simulink model "FOC"  (R2026a)
settings: Solver=FixedStepDiscrete  StopTime=inf  FixedStep=Ts  EnableMultiTasking=on
InitFcn:
  | ParameterInit
undefined symbols (not defined in the file): drive, FAKF, motor, Ts
libraries: mcbhdlcontrolslib x9, matrix_library x8, simulink x7, mcbcontrolslib x5, mcbsensorlessestimatorlib x2, mcbeeMathTransformLib x2, slpidlib x2, mcbpositiondecoderlib x1, sl_discontinuities x1
(part 1 of 2)
settings Model: Creator=xueji  LastModifiedBy=xuejf
settings DataIOCC: SaveFormat=StructureWithTime
settings OptimizationCC: ConditionallyExecuteInputs=off  UseDivisionForNetSlopeComputation=on  GainParamInheritBuiltInType=on  UseFloatMulNetSlope=on  StrengthReduction=on  NoFixptDivByZeroProtection=on  EfficientFloat2IntCast=on  OptimizationPriority=Speed  MultiThreadedLoops=on  AutoScheduleForLoops=on  UseRestrictQualifier=on
settings DebuggingCC: ParameterOverflowMsg=none  ParameterUnderflowMsg=error  ParameterPrecisionLossMsg=none
settings HardwareCC: ProdLargestAtomicInteger=Long  ProdLargestAtomicFloat=Double  ProdHWDeviceType=ARM Compatible->ARM Cortex  TargetBitPerPointer=64.0  TargetBitPerSizeT=64.0  TargetBitPerPtrDiffT=64.0  TargetLongLongMode=on  TargetIntDivRoundTo=Zero  TargetEndianess=LittleEndian  TargetWordSize=64.0  TargetHWDeviceType=MATLAB Host  ProdEqTarget=off
settings SFSimCC: SimTargetLang=C++
settings RTWCC: SystemTargetFile=ert.tlc  GenCodeOnly=on  Toolchain=GNU Tools for ARM Embedded Processors  BuildConfiguration=Faster Runs  DataTypeReplacement=CDataTypesFixedWidth  Description=Embedded Coder
settings CodeAppCC: CustomSymbolStrGlobalVar=rt$N$M  CustomSymbolStrType=$N$M  CustomSymbolStrFcn=$N$M$F  CustomSymbolStrMacro=$N$M  MATLABSourceComments=on  UseSimReservedNames=on
settings ERTTargetCC: ExtModeTransport=1.0  ExtModeMexFile=ext_serial_win32_comm  RootIOFormat=Structure reference  ERTFilePackagingFormat=Compact  MaxIdInt64=INT64_MAX  MinIdInt64=INT64_MIN  MaxIdUint64=UINT64_MAX  MaxIdInt32=INT32_MAX  MinIdInt32=INT32_MIN  MaxIdUint32=UINT32_MAX  MaxIdInt16=INT16_MAX  MinIdInt16=INT16_MIN  MaxIdUint16=UINT16_MAX  MaxIdInt8=INT8_MAX  MinIdInt8=INT8_MIN  MaxIdUint8=UINT8_MAX  GenerateSampleERTMain=on  CombineOutputUpdateFcns=off  SupportAbsoluteTime=off  PreserveMATLABNamespacesInGeneratedCode=off  CodeInterfacePackaging=Reusable function  SupportComplex=off
settings SimscapeCC: SimscapeNominalValues="[{\"value\":\"1\",\"unit\":\"A\"},{\"value\":\"1\",\"unit\":\"bar\"},{\"value\":\"1\",\"unit\":\"cm^2\"},{\"value\":\"1\",\"unit\":\"cm^3/s\"},{\"value\":\"1\",\"unit\":\"kJ/kg\"},{\"value\":\"1\",\"unit\":\"kW\"},{\"value\":\"1\",\"unit\":\"l\"},{\"value\":\"1\",\"unit\":\"N\"},{\"value\":\"1\",\"unit\":\"N*m\"},{\"value\":\"1\",\"unit\":\"V\"}]"  SimscapeLogType=none  SimscapeLogDataHistory=5000.0

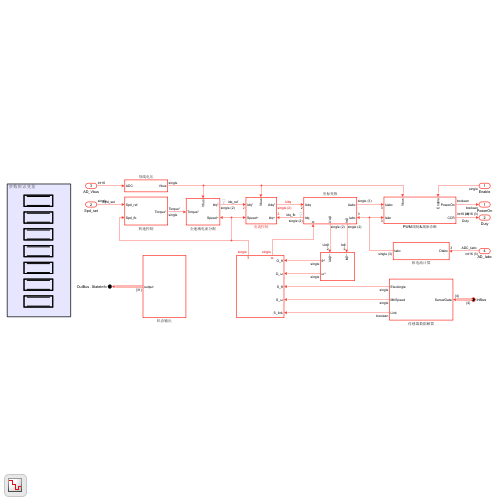
[thumbnail: Simulink's stored preview of the top-level diagram]
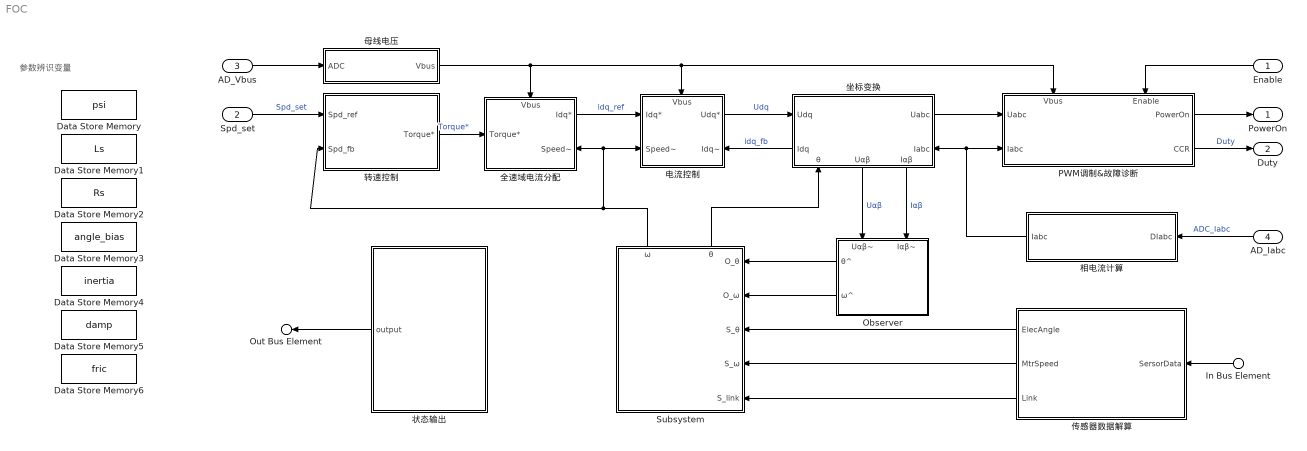
== system FOC ==
  note: 参数辨识变量
  Enable : Inport  OutDataTypeStr=single  PortDimensions=1  SampleTime=[5.0000000000000002e-05,0]
  Spd_set : Inport  Port=2  OutDataTypeStr=single  PortDimensions=1  SampleTime=[5.0000000000000002e-05,0]
  AD_Vbus : Inport  Port=3  OutDataTypeStr=int16  PortDimensions=1  SampleTime=[5.0000000000000002e-05,0]
  AD_Iabc : Inport  Port=4  OutDataTypeStr=int16  PortDimensions=3  SampleTime=[5.0000000000000002e-05,0]
  In Bus Element : Inport  Port=5  PortName=InBus
  Data Store Memory : DataStoreMemory  DataStoreName=psi  WriteAfterWriteMsg=warning  ShowAdditionalParam=off
  Data Store Memory1 : DataStoreMemory  DataStoreName=Ls  WriteAfterWriteMsg=warning  ShowAdditionalParam=off
  Data Store Memory2 : DataStoreMemory  DataStoreName=Rs  WriteAfterWriteMsg=warning  ShowAdditionalParam=off
  Data Store Memory3 : DataStoreMemory  DataStoreName=angle_bias  WriteAfterWriteMsg=warning  ShowAdditionalParam=off  OutDataTypeStr=single
  Data Store Memory4 : DataStoreMemory  DataStoreName=inertia  WriteAfterWriteMsg=warning  ShowAdditionalParam=off  OutDataTypeStr=single
  Data Store Memory5 : DataStoreMemory  DataStoreName=damp  WriteAfterWriteMsg=warning  ShowAdditionalParam=off  OutDataTypeStr=single
  Data Store Memory6 : DataStoreMemory  DataStoreName=fric  WriteAfterWriteMsg=warning  ShowAdditionalParam=off  OutDataTypeStr=single
  Observer : Subsystem
      settings: MinAlgLoopOccurrences=on  PortSchema="{\"entries\":[{\"content\":{\"sides\":[{\"content\":{\"connectorIds\":[\"Out1\",\"Out2\"]},\"type\":\"ConnectorPlacement.EquallySpacedRectSide\",\"uuid\":\"e0bc5786-ce1d-4855-a3b5-736cd4452aa5\"},{\"content\":{\"side\":\"RIGHT\"},\"type\":\"ConnectorPlacement.EquallySpacedRectSide\",\"uuid\":\"2fd42ec2-cdfa-4ba6-bbae-150322a5d493\"},{\"content\":{\"connectorIds\":[\"In1\",\"In2\"],\"side\":\"TOP\"},\"type\":\"ConnectorPlacement.EquallySpacedRectSide\",\"uuid\":\"b90c8681-3a82-4d31-b956-3e10c61bd992\"}]},\"type\":\"ConnectorPlacement.EquallySpacedConnector\",\"uuid\":\"5605c3b5-9268-4421-a61a-19e31e78b2b2\"}],\"packageUris\":[\"http://schema.mathworks.com/mf0/Connector/R2020b\"],\"version\":\"1.0\"}"
  PWM调制&故障诊断 : Subsystem
      settings: PortSchema="{\"entries\":[{\"content\":{\"sides\":[{\"content\":{\"connectorIds\":[\"In1\",\"In2\"]},\"type\":\"ConnectorPlacement.EquallySpacedRectSide\",\"uuid\":\"492d6452-e717-42c4-995f-3faa38429cae\"},{\"content\":{\"connectorIds\":[\"Out1\",\"Out2\"],\"side\":\"RIGHT\"},\"type\":\"ConnectorPlacement.EquallySpacedRectSide\",\"uuid\":\"a45b9f70-76fb-43db-a233-80127821733d\"},{\"content\":{\"connectorIds\":[\"In3\",\"In4\"],\"side\":\"TOP\"},\"type\":\"ConnectorPlacement.EquallySpacedRectSide\",\"uuid\":\"87480e42-0fd9-4078-9596-9cf4a8d8a61b\"},{\"content\":{\"side\":\"BOTTOM\"},\"type\":\"ConnectorPlacement.EquallySpacedRectSide\",\"uuid\":\"e85548a5-948a-4384-9ce6-748091ec18d7\"}]},\"type\":\"ConnectorPlacement.EquallySpacedConnector\",\"uuid\":\"18d7a9be-c392-4737-8548-f782ad0f8f26\"}],\"packageUris\":[\"http://schema.mathworks.com/mf0/Connector/R2020b\"],\"version\":\"1.0\"}"
  Subsystem : Subsystem
      settings: PortSchema="{\"entries\":[{\"content\":{\"sides\":[{\"content\":{},\"type\":\"ConnectorPlacement.EquallySpacedRectSide\",\"uuid\":\"d4a4fcc6-9eab-45aa-b231-b7af833cd8c6\"},{\"content\":{\"connectorIds\":[\"In1\",\"In2\",\"In3\",\"In4\",\"In5\"],\"side\":\"RIGHT\"},\"type\":\"ConnectorPlacement.EquallySpacedRectSide\",\"uuid\":\"bf374db6-391b-4179-b18d-5bc8f845fc33\"},{\"content\":{\"connectorIds\":[\"Out1\",\"Out2\"],\"side\":\"TOP\"},\"type\":\"ConnectorPlacement.EquallySpacedRectSide\",\"uuid\":\"b7b6826e-7c33-41ba-b3c7-d16a7d7beb3a\"}]},\"type\":\"ConnectorPlacement.EquallySpacedConnector\",\"uuid\":\"61c6cbd8-a55e-4c51-8b84-52df934ee1be\"}],\"packageUris\":[\"http://schema.mathworks.com/mf0/Connector/R2020b\"],\"version\":\"1.0\"}"
  传感器数据解算 : Subsystem
  全速域电流分配 : Subsystem
      settings: PortSchema="{\"entries\":[{\"content\":{\"sides\":[{\"content\":{\"connectorIds\":[\"In1\"]},\"type\":\"ConnectorPlacement.EquallySpacedRectSide\",\"uuid\":\"55c1d0af-1e12-4135-aa70-ca0befd6bb29\"},{\"content\":{\"connectorIds\":[\"Out1\",\"In3\"],\"side\":\"RIGHT\"},\"type\":\"ConnectorPlacement.EquallySpacedRectSide\",\"uuid\":\"d5856c39-d2d9-42bf-88a6-12c62f6eb837\"},{\"content\":{\"connectorIds\":[\"In2\"],\"side\":\"TOP\"},\"type\":\"ConnectorPlacement.EquallySpacedRectSide\",\"uuid\":\"f04465a3-695d-494e-bf21-7b8ba0e1a298\"}]},\"type\":\"ConnectorPlacement.EquallySpacedConnector\",\"uuid\":\"e6412d78-9d8b-45ef-81b3-23a4fb87ae10\"}],\"packageUris\":[\"http://schema.mathworks.com/mf0/Connector/R2020b\"],\"version\":\"1.0\"}"
  坐标变换 : Subsystem
      settings: PortSchema="{\"entries\":[{\"content\":{\"sides\":[{\"content\":{\"connectorIds\":[\"In1\",\"Out4\"]},\"type\":\"ConnectorPlacement.EquallySpacedRectSide\",\"uuid\":\"19423b74-9855-4da1-a32f-fc09d117de38\"},{\"content\":{\"connectorIds\":[\"Out1\",\"In3\"],\"side\":\"RIGHT\"},\"type\":\"ConnectorPlacement.EquallySpacedRectSide\",\"uuid\":\"45d897d7-b2dc-4681-bc4b-90a4bd929118\"},{\"content\":{\"connectorIds\":[],\"side\":\"TOP\"},\"type\":\"ConnectorPlacement.EquallySpacedRectSide\",\"uuid\":\"59354a96-0169-49af-a302-86e785c620a3\"},{\"content\":{\"connectorIds\":[\"In2\",\"Out2\",\"Out3\"],\"side\":\"BOTTOM\"},\"type\":\"ConnectorPlacement.EquallySpacedRectSide\",\"uuid\":\"fb332ee8-d153-4216-8303-19cfa3862110\"}]},\"type\":\"ConnectorPlacement.EquallySpacedConnector\",\"uuid\":\"5f6d72a6-e6b8-48f2-bb88-1ad3720f15b2\"}],\"packageUris\":[\"http://schema.mathworks.com/mf0/Connector/R2020b\"],\"version\":\"1.0\"}"
  母线电压 : Subsystem
  状态输出 : Subsystem
      settings: PortSchema="{\"entries\":[{\"content\":{\"sides\":[{\"content\":{\"connectorIds\":[\"Out1\"]},\"type\":\"ConnectorPlacement.EquallySpacedRectSide\",\"uuid\":\"5ecb5947-9baa-4bfe-8641-96ff20667d62\"},{\"content\":{\"side\":\"RIGHT\"},\"type\":\"ConnectorPlacement.EquallySpacedRectSide\",\"uuid\":\"3d186154-f081-4d30-a108-1a942147f536\"},{\"content\":{\"side\":\"TOP\"},\"type\":\"ConnectorPlacement.EquallySpacedRectSide\",\"uuid\":\"5aa511f5-28fe-4d78-8a7e-f2efec5693a1\"}]},\"type\":\"ConnectorPlacement.EquallySpacedConnector\",\"uuid\":\"ee06c015-bb25-435b-b725-56d91e20a522\"}],\"packageUris\":[\"http://schema.mathworks.com/mf0/Connector/R2020b\"],\"version\":\"1.0\"}"
  电流控制 : Subsystem
      settings: PortSchema="{\"entries\":[{\"content\":{\"sides\":[{\"content\":{\"connectorIds\":[\"In1\",\"In2\"]},\"type\":\"ConnectorPlacement.EquallySpacedRectSide\",\"uuid\":\"bf76b923-f33f-405a-8981-aa5371d2085f\"},{\"content\":{\"connectorIds\":[\"Out1\",\"In4\"],\"side\":\"RIGHT\"},\"type\":\"ConnectorPlacement.EquallySpacedRectSide\",\"uuid\":\"e7d4bdbe-138f-4605-8031-f7f1fbb983cf\"},{\"content\":{\"connectorIds\":[\"In3\"],\"side\":\"TOP\"},\"type\":\"ConnectorPlacement.EquallySpacedRectSide\",\"uuid\":\"9cdf7367-4fd9-4634-a6c3-b049cc73c34c\"},{\"content\":{\"side\":\"BOTTOM\"},\"type\":\"ConnectorPlacement.EquallySpacedRectSide\",\"uuid\":\"aba65895-d8a9-40f0-9a72-aa89d29f659a\"}]},\"type\":\"ConnectorPlacement.EquallySpacedConnector\",\"uuid\":\"3c2b3690-9a24-4e84-8e12-40b94ce0a856\"}],\"packageUris\":[\"http://schema.mathworks.com/mf0/Connector/R2020b\"],\"version\":\"1.0\"}"
  相电流计算 : Subsystem
  转速控制 : Subsystem
  PowerOn : Outport  OutDataTypeStr=boolean  PortDimensions=1  SampleTime=[5.0000000000000002e-05,0]
  Duty : Outport  Port=2  OutDataTypeStr=int16  PortDimensions=3  SampleTime=[5.0000000000000002e-05,0]
  Out Bus Element : Outport  Port=3  PortName=OutBus  Element=StateInfo
  wires:
  PWM调制&故障诊断/2(CCR) -> Duty/1  "Duty"
  坐标变换/4(Idq) -> 电流控制/4(Idq~)  "idq_fb"
  电流控制/1(Udq*) -> 坐标变换/1(Udq)  "Udq"
  坐标变换/1(Uabc) -> PWM调制&故障诊断/1(Uabc)
  Enable/1 -> PWM调制&故障诊断/4(Enable)
  坐标变换/2(Uαβ) -> Observer/1(Uαβ~)  "Uαβ"
  坐标变换/3(Iαβ) -> Observer/2(Iαβ~)  "Iαβ"
  Spd_set/1 -> 转速控制/1(Spd_ref)  "Spd_set"
  转速控制/1(Torque*) -> 全速域电流分配/1(Torque*)  "Torque*"
  全速域电流分配/1(Idq*) -> 电流控制/1(Idq*)  "idq_ref"
  相电流计算/1(Iabc) -> PWM调制&故障诊断/2(Iabc), 坐标变换/3(Iabc)
  PWM调制&故障诊断/1(PowerOn) -> PowerOn/1
  AD_Iabc/1 -> 相电流计算/1(DIabc)  "ADC_Iabc"
  母线电压/1(Vbus) -> 全速域电流分配/2(Vbus), 电流控制/3(Vbus), PWM调制&故障诊断/3(Vbus)
  AD_Vbus/1 -> 母线电压/1(ADC)
  传感器数据解算/2(MtrSpeed) -> Subsystem/4(S_ω)
  传感器数据解算/1(ElecAngle) -> Subsystem/3(S_θ)
  Subsystem/1(ω) -> 转速控制/2(Spd_fb), 全速域电流分配/3(Speed~), 电流控制/2(Speed~)
  Observer/1(θ^) -> Subsystem/1(O_θ)
  Subsystem/2(θ) -> 坐标变换/2(θ)
  Observer/2(ω^) -> Subsystem/2(O_ω)
  In Bus Element/1 -> 传感器数据解算/1(SersorData)
  状态输出/1(output) -> Out Bus Element/1
  传感器数据解算/3(Link) -> Subsystem/5(S_link)

== system FOC/Observer ==
  Uαβ~ : Inport
  Iαβ~ : Inport  Port=2
  AKF : Subsystem
  Demux : Demux  Outputs=2
  位置提取 : Subsystem
  对比观测器 : Subsystem  Commented=on
  角度转换 : Subsystem
  计算转子反电动势 : Subsystem
  转矩计算 : Subsystem
  θ^ : Outport
  ω^ : Outport  Port=2
  tag scope: Observer_Angle_e=global, Observer_Speed_m=global
  wires:
  Demux/2 -> 角度转换/1(θ), θ^/1, [Observer_Angle_e]
  AKF/1(x_k) -> Demux/1
  位置提取/1(ωθ) -> AKF/2(z_k)  "ωθ~"
  转矩计算/1(T) -> AKF/1(u_k)  "T"
  Iαβ~/1 -> 对比观测器/2(i), 转矩计算/2(I_αβ), 计算转子反电动势/1(Iαβ)
  计算转子反电动势/1(Eαβ) -> 位置提取/1(Eαβ)  "E_αβ"
  Uαβ~/1 -> 对比观测器/1(u), 计算转子反电动势/2(Uαβ)
  角度转换/1(sincos) -> 位置提取/2(θ_sincos), 转矩计算/1(θ_sincos)
  Demux/1 -> [Observer_Speed_m], ω^/1

== system FOC/PWM调制&故障诊断 ==
  Uabc : Inport
  Iabc : Inport  Port=2
  Vbus : Inport  Port=3
  Enable : Inport  Port=4
  Constant : Constant  Value=0.5  OutDataTypeStr=single
  Divide : Product  Inputs=*/
  Gain1 : Gain  Gain=drive.dead_time/drive.T_PWM  OutDataTypeStr=single
  Gain3 : Gain  Gain=drive.CNT_PWM  OutDataTypeStr=int16
  NOT : Logic  Operator=NOT  IconShape=distinctive  AllPortsSameDT=off  OutDataTypeStr=boolean
  NOT1 : Logic  IconShape=distinctive  AllPortsSameDT=off  OutDataTypeStr=boolean
  Sign : Signum
  Sum : Sum  Inputs=+++
  故障诊断 : Subsystem
  限幅1 : Saturate  UpperLimit=drive.CNT_PWM*0.99  LowerLimit=drive.CNT_PWM*0.01
  PowerOn : Outport
  CCR : Outport  Port=2
  tag scope: U_bus=global
  wires:
  Gain3/1 -> 限幅1/1
  Vbus/1 -> 故障诊断/2(U_bus), Divide/2, [U_bus]
  Sum/1 -> Gain3/1
  Constant/1 -> Sum/3
  NOT1/1 -> PowerOn/1
  故障诊断/1(Err_code) -> NOT/1
  Enable/1 -> NOT1/2
  NOT/1 -> NOT1/1
  Gain1/1 -> Sum/1
  Iabc/1 -> Sign/1, 故障诊断/1(I_abc)
  Sign/1 -> Gain1/1
  限幅1/1 -> CCR/1
  Uabc/1 -> Divide/1
  Divide/1 -> Sum/2  "Duty"

== system FOC/Subsystem ==
  O_θ : Inport
  O_ω : Inport  Port=2
  S_θ : Inport  Port=3
  S_ω : Inport  Port=4
  S_link : Inport  Port=5
  Switch : Switch  Criteria=u2 > Threshold  SaturateOnIntegerOverflow=off  InputSameDT=off
  Switch1 : Switch  Criteria=u2 > Threshold  SaturateOnIntegerOverflow=off  InputSameDT=off
  ω : Outport
  θ : Outport  Port=2
  wires:
  Switch1/1 -> ω/1
  Switch/1 -> θ/1
  S_link/1 -> Switch/2, Switch1/2
  S_ω/1 -> Switch1/1
  O_θ/1 -> Switch/3
  S_θ/1 -> Switch/1
  O_ω/1 -> Switch1/3

== system FOC/传感器数据解算 ==
  SersorData : Inport
  Bus Selector2 : BusSelector  OutputSignals=Hall,Encoder
  Terminator : Terminator
  角度计算 : Subsystem
  转速计算 : Subsystem
  ElecAngle : Outport
  MtrSpeed : Outport  Port=2
  Link : Outport  Port=3
  tag scope: Sensor_Angle_e=global, Sensor_Speed_m=global
  wires:
  角度计算/3(Link) -> Link/1
  角度计算/2(ElecAngle) -> ElecAngle/1, [Sensor_Angle_e]
  Bus Selector2/1 -> 角度计算/1(Hall)  "<Hall>"
  Bus Selector2/2 -> 角度计算/2(Encoder), 转速计算/1(Encoder)  "<Encoder>"
  转速计算/1(MtrSpeed) -> MtrSpeed/1, [Sensor_Speed_m]
  角度计算/1(MtrPos) -> Terminator/1
  SersorData/1 -> Bus Selector2/1

== system FOC/全速域电流分配 ==
  Torque* : Inport
  Vbus : Inport  Port=2
  Speed~ : Inport  Port=3
  Constant1 : Constant  Value=motor.I_max  OutDataTypeStr=single
  Gain : Gain  Gain=1/motor.Kt
  Gain2 : Gain  Gain=-1
  IIR Filter1 : mcbhdlcontrolslib/IIR Filter  VariantControl=Low Pass Filter  VariantSelect=Low-pass  FilterConstantInputType=Specify via dialog  Filter_constant=0.1  advancedSettings=off  Ts=50e-6  cutOff_freq=353.6777
  MJPA : Subsystem
  Math Function : Math  Operator=square
  Math Function1 : Math  Operator=square
  Mux1 : Mux  Inputs=2
  Saturation Dynamic : sl_discontinuities/Saturation Dynamic  OutMin=[]  OutMax=[]  OutDataTypeStr=single  OutDataType=fixdt(1, 16)  OutScaling=2^-10  DoSatur=off
  Sqrt : Sqrt
  Sum1 : Sum  Inputs=-+|
  Idq* : Outport
  tag scope: Speed_m=global
  wires:
  Gain/1 -> Saturation Dynamic/2
  IIR Filter1/1 -> Idq*/1
  Math Function1/1 -> Sum1/2
  MJPA/1(i*_d) -> Mux1/1, Math Function/1
  Vbus/1 -> MJPA/1(Vbus)
  Gain2/1 -> Saturation Dynamic/3
  Sqrt/1 -> Saturation Dynamic/1, Gain2/1
  Sum1/1 -> Sqrt/1
  Math Function/1 -> Sum1/1
  Constant1/1 -> Math Function1/1
  Speed~/1 -> [Speed_m], MJPA/2(ω_m)
  Torque*/1 -> Gain/1
  Mux1/1 -> IIR Filter1/1
  Saturation Dynamic/1 -> Mux1/2

== system FOC/坐标变换 ==
  Udq : Inport
  θ : Inport  Port=2
  Iabc : Inport  Port=3
  Subsystem11 : Subsystem
  Subsystem2 : Subsystem
      settings: PortSchema="{\"entries\":[{\"content\":{\"sides\":[{\"content\":{\"connectorIds\":[\"In1\"]},\"type\":\"ConnectorPlacement.EquallySpacedRectSide\",\"uuid\":\"492d6452-e717-42c4-995f-3faa38429cae\"},{\"content\":{\"connectorIds\":[\"Out1\"],\"side\":\"RIGHT\"},\"type\":\"ConnectorPlacement.EquallySpacedRectSide\",\"uuid\":\"a45b9f70-76fb-43db-a233-80127821733d\"},{\"content\":{\"connectorIds\":[\"In2\"],\"side\":\"TOP\"},\"type\":\"ConnectorPlacement.EquallySpacedRectSide\",\"uuid\":\"87480e42-0fd9-4078-9596-9cf4a8d8a61b\"},{\"content\":{\"connectorIds\":[],\"side\":\"BOTTOM\"},\"type\":\"ConnectorPlacement.EquallySpacedRectSide\",\"uuid\":\"abbb6dc7-6c8b-4aee-9a22-efe0eeab5972\"}]},\"type\":\"ConnectorPlacement.EquallySpacedConnector\",\"uuid\":\"18d7a9be-c392-4737-8548-f782ad0f8f26\"}],\"packageUris\":[\"http://schema.mathworks.com/mf0/Connector/R2020b\"],\"version\":\"1.0\"}"
  Subsystem3 : Subsystem
  Subsystem4 : Subsystem
  Subsystem5 : Subsystem
      settings: PortSchema="{\"entries\":[{\"content\":{\"sides\":[{\"content\":{\"connectorIds\":[\"In1\"]},\"type\":\"ConnectorPlacement.EquallySpacedRectSide\",\"uuid\":\"492d6452-e717-42c4-995f-3faa38429cae\"},{\"content\":{\"connectorIds\":[\"Out1\"],\"side\":\"RIGHT\"},\"type\":\"ConnectorPlacement.EquallySpacedRectSide\",\"uuid\":\"a45b9f70-76fb-43db-a233-80127821733d\"},{\"content\":{\"connectorIds\":[],\"side\":\"TOP\"},\"type\":\"ConnectorPlacement.EquallySpacedRectSide\",\"uuid\":\"87480e42-0fd9-4078-9596-9cf4a8d8a61b\"},{\"content\":{\"connectorIds\":[\"In2\"],\"side\":\"BOTTOM\"},\"type\":\"ConnectorPlacement.EquallySpacedRectSide\",\"uuid\":\"c5a9fd10-4005-478b-ab9c-ebed3c1e9985\"}]},\"type\":\"ConnectorPlacement.EquallySpacedConnector\",\"uuid\":\"18d7a9be-c392-4737-8548-f782ad0f8f26\"}],\"packageUris\":[\"http://schema.mathworks.com/mf0/Connector/R2020b\"],\"version\":\"1.0\"}"
  Uabc : Outport
  Uαβ : Outport  Port=2
  Iαβ : Outport  Port=3
  Idq : Outport  Port=4
  tag scope: I_abc=global, U_abc=global
  wires:
  Iabc/1 -> [I_abc], Subsystem3/1(abc)
  Subsystem4/1(abc) -> [U_abc], Uabc/1
  θ/1 -> Subsystem11/1(angle)  "E_angle"
  Subsystem2/1(dq) -> Idq/1  "Idq_fb"
  Subsystem3/1(αβ) -> Subsystem2/1(αβ), Iαβ/1  "Iαβ"
  Subsystem5/1(αβ) -> Subsystem4/1(αβ), Uαβ/1  "Uαβ"
  Subsystem11/1(sincos) -> Subsystem5/2(sincos), Subsystem2/2(sincos)
  Udq/1 -> Subsystem5/1(dq)

== system FOC/母线电压 ==
  ADC : Inport
  Gain : Gain  Gain=drive.ADC_Vref/(drive.V_gain*drive.ADC_MaxCount*2)  OutDataTypeStr=single
  母线电压采样滤波 : mcbhdlcontrolslib/IIR Filter  VariantControl=Low Pass Filter  VariantSelect=Low-pass  FilterConstantInputType=Specify via dialog  Filter_constant=0.1  advancedSettings=off  Ts=50e-6  cutOff_freq=353.6777
  Vbus : Outport
  wires:
  ADC/1 -> Gain/1
  母线电压采样滤波/1 -> Vbus/1
  Gain/1 -> 母线电压采样滤波/1

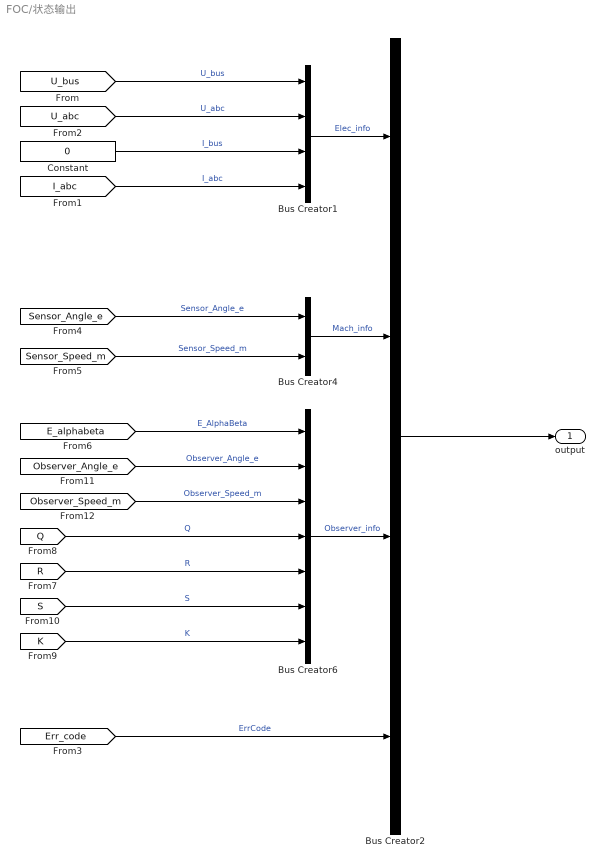
== system FOC/状态输出 ==
  Bus Creator1 : BusCreator  Inputs=4
  Bus Creator2 : BusCreator  Inputs=4
  Bus Creator4 : BusCreator  Inputs=2
  Bus Creator6 : BusCreator  Inputs=7
  Constant : Constant  Value=0  OutDataTypeStr=single
  output : Outport
  wires:
  Bus Creator6/1 -> Bus Creator2/3  "Observer_info"
  [Observer_Speed_m] -> Bus Creator6/3  "Observer_Speed_m"
  [Observer_Angle_e] -> Bus Creator6/2  "Observer_Angle_e"
  [E_alphabeta] -> Bus Creator6/1  "E_AlphaBeta"
  [Err_code] -> Bus Creator2/4  "ErrCode"
  [K] -> Bus Creator6/7  "K"
  [S] -> Bus Creator6/6  "S"
  [R] -> Bus Creator6/5  "R"
  [Q] -> Bus Creator6/4  "Q"
  [U_abc] -> Bus Creator1/2  "U_abc"
  Bus Creator4/1 -> Bus Creator2/2  "Mach_info"
  Bus Creator1/1 -> Bus Creator2/1  "Elec_info"
  Constant/1 -> Bus Creator1/3  "I_bus"
  [Sensor_Speed_m] -> Bus Creator4/2  "Sensor_Speed_m"
  [Sensor_Angle_e] -> Bus Creator4/1  "Sensor_Angle_e"
  Bus Creator2/1 -> output/1
  [I_abc] -> Bus Creator1/4  "I_abc"
  [U_bus] -> Bus Creator1/1  "U_bus"

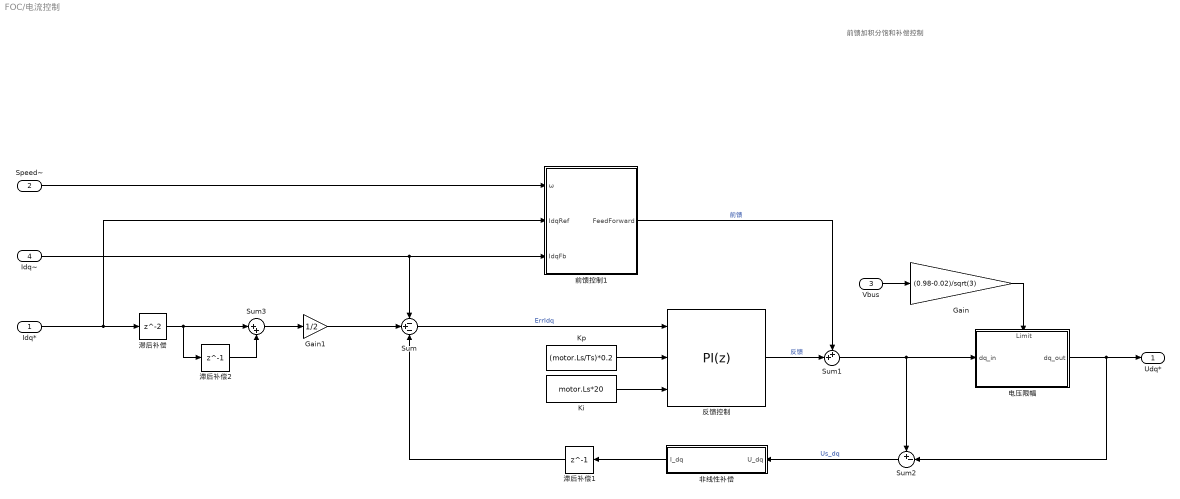
== system FOC/电流控制 ==
  note: 前馈加积分饱和补偿控制
  Idq* : Inport
  Speed~ : Inport  Port=2
  Vbus : Inport  Port=3
  Idq~ : Inport  Port=4
  Gain : Gain  Gain=(0.98-0.02)/sqrt(3)
  Gain1 : Gain  Gain=1/2
  Ki : Constant  Value=motor.Ls*20  OutDataTypeStr=single  SampleTime=-1
  Kp : Constant  Value=(motor.Ls/Ts)*0.2  OutDataTypeStr=single  SampleTime=-1
  Sum : Sum  Inputs=-+-
  Sum1 : Sum  Inputs=++|
  Sum2 : Sum  Inputs=+-|
  Sum3 : Sum  Inputs=|++
  前馈控制1 : Subsystem
  反馈控制 : slpidlib/PID Controller  Controller=PI  Form=Parallel  TimeDomain=Discrete-time  UseExternalTs=off  SampleTime=-1  IntegratorMethod=Forward Euler  FilterMethod=Forward Euler  ControllerParametersSource=external  P=1  I=1  UseKiTs=on  D=0  UseExternalDerivativeSource=off  N=100  UseFilter=on  TunerSelectOption=Transfer Function Based (PID Tuner App)  InitialConditionSource=internal  InitialConditionForIntegrator=0  InitialConditionForFilter=0  DifferentiatorICPrevScaledInput=0  ExternalReset=none  TrackingMode=off  Kt=1  LimitOutput=off  SatLimitsSource=internal  UpperSaturationLimit=drive.V_bus/2  LowerSaturationLimit=-drive.V_bus/2  LinearizeAsGain=on  AntiWindupMode=clamping  Kb=1  LimitIntegrator=off  UpperIntegratorSaturationLimit=inf  LowerIntegratorSaturationLimit=-inf  RndMeth=Simplest  POutMin=[]  POutMax=[]  IOutMin=[]  IOutMax=[]  DOutMin=[]  DOutMax=[]  NOutMin=[]  NOutMax=[]  SumOutMin=[]  SumOutMax=[]  SaturationOutDataTypeStr=Inherit: Inherit via back propagation  SaturationOutMin=[]  SaturationOutMax=[]  PParamMin=[]  PParamMax=[]  IParamMin=[]  IParamMax=[]  DParamMin=[]  DParamMax=[]  NParamMin=[]  NParamMax=[]  KbParamMin=[]  KbParamMax=[]  KtParamMin=[]  KtParamMax=[]  KbOutMin=[]  KbOutMax=[]  KtOutMin=[]  KtOutMax=[]  IntegratorOutMin=[]  IntegratorOutMax=[]  FilterOutMin=[]  FilterOutMax=[]  SumI1OutMin=[]  SumI1OutMax=[]  SumI2OutMin=[]  SumI2OutMax=[]  SumI3OutMin=[]  SumI3OutMax=[]  SumI4OutMin=[]  SumI4OutMax=[]  SumDOutMin=[]  SumDOutMax=[]  DifferentiatorOutMin=[]  DifferentiatorOutMax=[]  FilterDiffOutCoefMin=[]  FilterDiffOutCoefMax=[]  ReciprocalOutMin=[]  ReciprocalOutMax=[]  SumDenOutMin=[]  SumDenOutMax=[]  SumNumOutMin=[]  SumNumOutMax=[]  DivideOutMin=[]  DivideOutMax=[]  UdiffTsProdOutMin=[]  UdiffTsProdOutMax=[]  NTsProdOutMin=[]  NTsProdOutMax=[]  UintegralTsProdOutMin=[]  UintegralTsProdOutMax=[]  UngainTsProdOutMin=[]  UngainTsProdOutMax=[]  ClampingZeroOutDataTypeStr=Inherit: Inherit via back propagation  ClampingZeroOutMin=[]  ClampingZeroOutMax=[]  FilterDenConstantOutDataTypeStr=Inherit: Inherit via back propagation  FilterDenConstantOutMin=[]  FilterDenConstantOutMax=[]  PCopyOutDataTypeStr=Inherit: Inherit via back propagation  PCopyOutMin=[]  PCopyOutMax=[]  NCopyOutDataTypeStr=Inherit: Inherit via back propagation  NCopyOutMin=[]  NCopyOutMax=[]  IntegratorContinuousStateAttributes=''  IntegratorStateMustResolveToSignalObject=off  IntegratorRTWStateStorageClass=Auto  FilterContinuousStateAttributes=''  FilterStateMustResolveToSignalObject=off  FilterRTWStateStorageClass=Auto  ParallelPVariant=ExternalParameters  IdealPVariant=Disabled  IVariant=ExternalParameters  DVariant=Disabled  IntegratorVariant=Discrete  SatVariant=Disabled  AWVariant=Passthrough  PCopyVariant=Disabled  TRVariant=Disabled  FdbkBlocksVariant=Forward  IdealPFdbkVariant=Disabled  SatFdbkVariant=Disabled  DerivativeFilterVariant=Disabled  NVariant=Disabled  NCopyVariant=Disabled_SignalSpec  FilterICVariant=Disabled  IntegratorICVariant=InternalICs  ExternalResetVariant=Disabled  TRSumVariant=Passthrough  SumFdbkVariant=Disabled  SumVariant=Sum_PI  TsampFilterVariant=InternalTs  TsampNgainVariant=Passthrough  TsampIntegralVariant=Disabled_SignalSpec  ExternalSaturationOutDataTypeStr=Inherit: Same as second input  DerivativeSourceVariant=Disabled  PreIntVariant=InternalPreInt
  滞后补偿 : Delay
  滞后补偿1 : Delay  DelayLength=1
  滞后补偿2 : Delay  DelayLength=1
  电压限幅 : Subsystem
      settings: PortSchema="{\"entries\":[{\"content\":{\"sides\":[{\"content\":{\"connectorIds\":[\"In1\"]},\"type\":\"ConnectorPlacement.EquallySpacedRectSide\",\"uuid\":\"8318c52a-9d90-468d-b9ba-7dc43530864a\"},{\"content\":{\"connectorIds\":[\"Out1\"],\"side\":\"RIGHT\"},\"type\":\"ConnectorPlacement.EquallySpacedRectSide\",\"uuid\":\"ec35b037-8c54-4ea5-a44f-2157489f6ede\"},{\"content\":{\"connectorIds\":[\"In2\"],\"side\":\"TOP\"},\"type\":\"ConnectorPlacement.EquallySpacedRectSide\",\"uuid\":\"86589762-ebe7-4f54-bef4-fc17ac715e1b\"}]},\"type\":\"ConnectorPlacement.EquallySpacedConnector\",\"uuid\":\"5c9fe270-4db2-4b15-bc03-dab13b772a86\"}],\"packageUris\":[\"http://schema.mathworks.com/mf0/Connector/R2020b\"],\"version\":\"1.0\"}"
  非线性补偿 : Subsystem
  Udq* : Outport  VectorParamsAs1DForOutWhenUnconnected=off
  wires:
  滞后补偿1/1 -> Sum/3
  Idq*/1 -> 前馈控制1/2(IdqRef), 滞后补偿/1
  前馈控制1/1(FeedForward) -> Sum1/1  "前馈"
  Sum1/1 -> 电压限幅/1(dq_in), Sum2/1
  Gain1/1 -> Sum/2
  Sum3/1 -> Gain1/1
  滞后补偿2/1 -> Sum3/2
  非线性补偿/1(I_dq) -> 滞后补偿1/1
  Sum2/1 -> 非线性补偿/1(U_dq)  "Us_dq"
  Gain/1 -> 电压限幅/2(Limit)
  Speed~/1 -> 前馈控制1/1(ω)
  电压限幅/1(dq_out) -> Udq*/1, Sum2/2
  Vbus/1 -> Gain/1
  滞后补偿/1 -> 滞后补偿2/1, Sum3/1
  Kp/1 -> 反馈控制/2
  Ki/1 -> 反馈控制/3
  Idq~/1 -> Sum/1, 前馈控制1/3(IdqFb)
  Sum/1 -> 反馈控制/1  "ErrIdq"
  反馈控制/1 -> Sum1/2  "反馈"

== system FOC/相电流计算 ==
  DIabc : Inport
  DA转换 : Gain  Gain=drive.ADC_Vref/(drive.ADC_MaxCount*2)  OutDataTypeStr=single
  Data Type Conversion : DataTypeConversion  OutDataTypeStr=single  SaturateOnIntegerOverflow=off  RndMeth=Floor
  Gain1 : Gain  Gain=1/3
  Sum : Sum  Inputs=|+-
  Sum of Elements : Sum  Inputs=+
  电流计算 : Gain  Gain=1/drive.I_gain
  Iabc : Outport
  wires:
  电流计算/1 -> Sum of Elements/1, Sum/1
  Sum of Elements/1 -> Gain1/1
  Gain1/1 -> Sum/2
  Sum/1 -> Iabc/1
  Data Type Conversion/1 -> DA转换/1
  DIabc/1 -> Data Type Conversion/1
  DA转换/1 -> 电流计算/1  "电压"

== system FOC/转速控制 ==
  Spd_ref : Inport
  Spd_fb : Inport  Port=2
  Constant : Constant  Value=0.015  OutDataTypeStr=single
  Constant1 : Constant  Value=0.2*Ts  OutDataTypeStr=single
  Constant3 : Constant  Value=0  OutDataTypeStr=single
  Math Function1 : Math  Operator=square
  Math Function2 : Math  Operator=square
  Math Function3 : Math  Operator=square
  PI控制器 : slpidlib/PID Controller  Controller=PI  Form=Parallel  TimeDomain=Discrete-time  UseExternalTs=off  SampleTime=Ts  IntegratorMethod=Forward Euler  FilterMethod=Forward Euler  ControllerParametersSource=external  P=1  I=1  UseKiTs=on  D=0  UseExternalDerivativeSource=off  N=100  UseFilter=on  TunerSelectOption=Transfer Function Based (PID Tuner App)  InitialConditionSource=external  InitialConditionForIntegrator=0  InitialConditionForFilter=0  DifferentiatorICPrevScaledInput=0  ExternalReset=level  TrackingMode=off  Kt=1  LimitOutput=on  SatLimitsSource=internal  UpperSaturationLimit=motor.T_rated  LowerSaturationLimit=-motor.T_rated  LinearizeAsGain=on  AntiWindupMode=clamping  Kb=1  LimitIntegrator=off  UpperIntegratorSaturationLimit=inf  LowerIntegratorSaturationLimit=-inf  RndMeth=Simplest  POutMin=[]  POutMax=[]  IOutMin=[]  IOutMax=[]  DOutMin=[]  DOutMax=[]  NOutMin=[]  NOutMax=[]  SumOutMin=[]  SumOutMax=[]  SaturationOutDataTypeStr=Inherit: Inherit via back propagation  SaturationOutMin=[]  SaturationOutMax=[]  PParamMin=[]  PParamMax=[]  IParamMin=[]  IParamMax=[]  DParamMin=[]  DParamMax=[]  NParamMin=[]  NParamMax=[]  KbParamMin=[]  KbParamMax=[]  KtParamMin=[]  KtParamMax=[]  KbOutMin=[]  KbOutMax=[]  KtOutMin=[]  KtOutMax=[]  IntegratorOutMin=[]  IntegratorOutMax=[]  FilterOutMin=[]  FilterOutMax=[]  SumI1OutMin=[]  SumI1OutMax=[]  SumI2OutMin=[]  SumI2OutMax=[]  SumI3OutMin=[]  SumI3OutMax=[]  SumI4OutMin=[]  SumI4OutMax=[]  SumDOutMin=[]  SumDOutMax=[]  DifferentiatorOutMin=[]  DifferentiatorOutMax=[]  FilterDiffOutCoefMin=[]  FilterDiffOutCoefMax=[]  ReciprocalOutMin=[]  ReciprocalOutMax=[]  SumDenOutMin=[]  SumDenOutMax=[]  SumNumOutMin=[]  SumNumOutMax=[]  DivideOutMin=[]  DivideOutMax=[]  UdiffTsProdOutMin=[]  UdiffTsProdOutMax=[]  NTsProdOutMin=[]  NTsProdOutMax=[]  UintegralTsProdOutMin=[]  UintegralTsProdOutMax=[]  UngainTsProdOutMin=[]  UngainTsProdOutMax=[]  ClampingZeroOutDataTypeStr=Inherit: Inherit via back propagation  ClampingZeroOutMin=[]  ClampingZeroOutMax=[]  FilterDenConstantOutDataTypeStr=Inherit: Inherit via back propagation  FilterDenConstantOutMin=[]  FilterDenConstantOutMax=[]  PCopyOutDataTypeStr=Inherit: Inherit via back propagation  PCopyOutMin=[]  PCopyOutMax=[]  NCopyOutDataTypeStr=Inherit: Inherit via back propagation  NCopyOutMin=[]  NCopyOutMax=[]  IntegratorContinuousStateAttributes=''  IntegratorStateMustResolveToSignalObject=off  IntegratorRTWStateStorageClass=Auto  FilterContinuousStateAttributes=''  FilterStateMustResolveToSignalObject=off  FilterRTWStateStorageClass=Auto  ParallelPVariant=ExternalParameters  IdealPVariant=Disabled  IVariant=ExternalParameters  DVariant=Disabled  IntegratorVariant=Discrete  SatVariant=Enabled  AWVariant=DiscClampingParallel  PCopyVariant=Disabled  TRVariant=Disabled  FdbkBlocksVariant=Forward  IdealPFdbkVariant=Disabled  SatFdbkVariant=Disabled  DerivativeFilterVariant=Disabled  NVariant=Disabled  NCopyVariant=Disabled_SignalSpec  FilterICVariant=Disabled  IntegratorICVariant=ExternalICs  ExternalResetVariant=ExternalReset  TRSumVariant=Passthrough  SumFdbkVariant=Disabled  SumVariant=Sum_PI  TsampFilterVariant=InternalTs  TsampNgainVariant=Passthrough  TsampIntegralVariant=Disabled_SignalSpec  ExternalSaturationOutDataTypeStr=Inherit: Same as second input  DerivativeSourceVariant=Disabled  PreIntVariant=InternalPreInt
  Saturation1 : Saturate  UpperLimit=motor.radps_max  LowerLimit=-motor.radps_max
  Sum : Sum  Inputs=|+-
  Sum1 : Sum  Inputs=++|
  判断 : RelationalOperator  Operator=<  OutDataTypeStr=boolean  RndMeth=Simplest  InputSameDT=off
  额定转速2% : Constant  Value=motor.radps_rated*0.00  OutDataTypeStr=single
  Torque* : Outport
  wires:
  Math Function3/1 -> 判断/2
  Constant3/1 -> PI控制器/5
  额定转速2%/1 -> Math Function3/1
  判断/1 -> PI控制器/4
  Sum1/1 -> 判断/1
  Math Function1/1 -> Sum1/1
  Math Function2/1 -> Sum1/2
  Saturation1/1 -> Sum/1, Math Function1/1
  Constant1/1 -> PI控制器/3
  Spd_ref/1 -> Saturation1/1
  Spd_fb/1 -> Sum/2, Math Function2/1
  Sum/1 -> PI控制器/1
  PI控制器/1 -> Torque*/1  "扭矩"
  Constant/1 -> PI控制器/2

== system FOC/Observer/AKF ==
  u_k : Inport
  z_k : Inport  Port=2
  协方差估计 : Subsystem
  协方差计算 : Subsystem
  状态观测 : Subsystem
  x_k : Outport
  tag scope: K=global, Q=global, R=global, S=global, T=global
  wires:
  协方差计算/3(T) -> 协方差估计/4(T), [T]  "T"
  协方差计算/1(K) -> 状态观测/3(K), [K]  "K"
  协方差估计/2(Q) -> 协方差计算/2(Q), [Q]  "Q"
  协方差计算/2(S) -> 协方差估计/3(S), [S]  "S"
  状态观测/2(e~) -> 协方差估计/1(e~)  "e~"
  状态观测/3(e^) -> 协方差估计/2(e^)  "e^"
  状态观测/1(x^) -> x_k/1  "x^"
  z_k/1 -> 状态观测/2(z)
  u_k/1 -> 状态观测/1(u)
  协方差估计/1(R) -> [R], 协方差计算/1(R)  "R"

== system FOC/Observer/位置提取 ==
  Eαβ : Inport
  θ_sincos : Inport  Port=2
  Constant : Constant  Value=motor.psi  OutDataTypeStr=single
  Demux : Demux  Outputs=2
  Divide3 : Product  Inputs=/*
  Gain : Gain  Gain=[-1 1]  Multiplication=Matrix(K*u)
  Gain1 : Gain  Gain=motor.P
  Gain2 : Gain  Gain=-1
  Mux : Mux  Inputs=2
  Product : Product
  Product1 : Product
  Sign : Signum
  Unit Delay : UnitDelay  SampleTime=-1
  幅角 : mcbcontrolslib/atan2  ApproximationMethod=None  NumberOfIterations=11  NumberOfDataPoints=16  InterpMethod=Flat  outputUnit=Radians  TableDataTypeStr=Inherit: Inherit via input
  ωθ : Outport
  wires:
  Product1/1 -> Demux/1
  Sign/1 -> Product1/1
  Eαβ/1 -> Product1/2, Product/2
  Gain2/1 -> 幅角/1
  Demux/1 -> Gain2/1
  Demux/2 -> 幅角/2
  Mux/1 -> ωθ/1
  Divide3/1 -> Mux/1
  Gain/1 -> Sign/1, Divide3/2
  Product/1 -> Gain/1
  Unit Delay/1 -> Product/1
  θ_sincos/1 -> Unit Delay/1
  幅角/1 -> Mux/2
  Gain1/1 -> Divide3/1
  Constant/1 -> Gain1/1

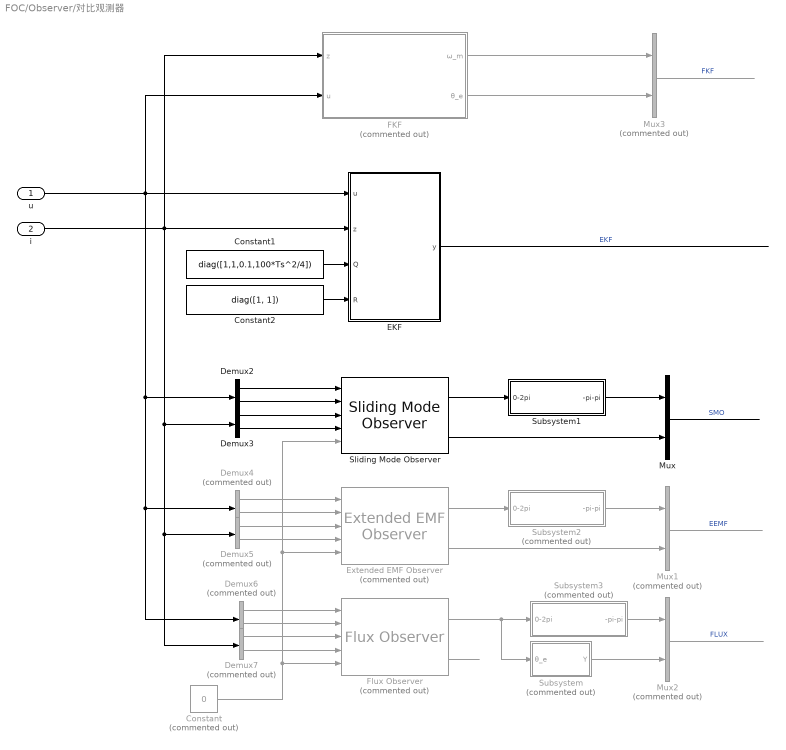
== system FOC/Observer/对比观测器 ==
  u : Inport
  i : Inport  Port=2
  Constant : Constant  Commented=on  Value=0  OutDataTypeStr=single
  Constant1 : Constant  Value=diag([1,1,0.1,100*Ts^2/4])  OutDataTypeStr=single
  Constant2 : Constant  Value=diag([1, 1])  OutDataTypeStr=single
  Demux2 : Demux  Outputs=2
  Demux3 : Demux  Outputs=2
  Demux{4..7} (4 alike) : Demux  Commented=on  Outputs=2
  EKF : Subsystem
  Extended EMF Observer : mcbsensorlessestimatorlib/Extended EMF Observer  Commented=on  ParameterBusInput=off  InputUnit=SI unit  PosOut=Electrical position  BlkSampleTime=Ts  MotorSelection=PMSM  EEMFMultiplier=10  StatorResistance=motor.Rs  StatorDaxisInductance=motor.Ls  StatorQaxisInductance=motor.Ls  MaxApplicationSpeed=3000  PolePairs=motor.P  MaxStatorVoltage=12*sqrt(3)  MaxStatorCurrent=10  Alpha=50  EEMFCutoffFreq=50  Kp=250  Ki=200000  N_points=1024  SpeedCutoffFreq=50  PositionUnit=Radians  PositionDataType=single  SpeedUnit=Radians/sec  PerUnitSpeed=6000  SpeedDataType=single  TableDatatype=single
      settings: LibrarySourceBlock=mcblib/Sensorless Estimators/Extended EMF Observer
  FKF : Subsystem  Commented=on
  Flux Observer : mcbpositiondecoderlib/Flux Observer  Commented=on  DataTypeSelect=off  ParameterBusInput=off  MotorSelection=PMSM  BlockInputUnit=Per-unit  PerUnitVoltage=12*sqrt(3)  PerUnitCurrent=10  PositionSelect=on  FluxSelect=off  TorqueSelect=on  PolePairs=4  StatorResistance=0.36  StatorDAxisInductance=0.2e-3  StatorLeakageInductance=0.0068  RotorLeakageInductance=0.0068  MagnetizingInductance=0.0300  CutoffFreq=50  BlockSampleTime=Ts  PositionUnit=Radians  PositionDatatype=single  FluxUnit=Weber  PerUnitFlux=0.1  FluxDatatype=single  TorqueUnit=Nm  PerUnitTorque=100  TorqueDatatype=single  DataType=0
      settings: LibrarySourceBlock=mcblib/Sensorless Estimators/Flux Observer
  Mux : Mux  Inputs=2
  Mux1 : Mux  Commented=on  Inputs=2
  Mux2 : Mux  Commented=on  Inputs=2
  Mux3 : Mux  Commented=on  Inputs=2
  Sliding Mode Observer : mcbsensorlessestimatorlib/Sliding Mode Observer  InputUnit=Per-unit  BlkSampleTime=Ts  StatorResistance=motor.Rs  StatorInductance=motor.Ls  MaxApplicationSpeed=3000  PolePairs=motor.P  MaxStatorVoltage=12*sqrt(3)  MaxStatorCurrent=10  DisturbanceObserverGain=0.9  CurrentObserverGain=0.5  CutoffFreq=600  PositionUnit=Radians  PositionDataType=single  SpeedUnit=Radians/sec  PerUnitSpeed=6000  SpeedDataType=single
      settings: LibrarySourceBlock=mcblib/Sensorless Estimators/Sliding Mode Observer
  Subsystem : Subsystem  Commented=on
  Subsystem1 : Subsystem
  Subsystem2 : Subsystem  Commented=on
  Subsystem3 : Subsystem  Commented=on
  wires:
  Subsystem3/1(-pi-pi) -> Mux2/1
  Subsystem2/1(-pi-pi) -> Mux1/1
  Subsystem1/1(-pi-pi) -> Mux/1
  Mux3/1 -> ?  "FKF"
  FKF/2(θ_e) -> Mux3/2
  FKF/1(ω_m) -> Mux3/1
  Mux2/1 -> ?  "FLUX"
  Mux1/1 -> ?  "EEMF"
  Mux/1 -> ?  "SMO"
  Subsystem/1(Y) -> Mux2/2
  EKF/1(y) -> ?  "EKF"
  i/1 -> EKF/2(z), FKF/1(z), Demux7/1, Demux5/1, Demux3/1
  Constant1/1 -> EKF/3(Q)
  Constant2/1 -> EKF/4(R)
  u/1 -> Demux6/1, Demux4/1, Demux2/1, FKF/2(u), EKF/1(u)
  Demux4/2 -> Extended EMF Observer/2
  Demux4/1 -> Extended EMF Observer/1
  Demux5/1 -> Extended EMF Observer/3
  Demux5/2 -> Extended EMF Observer/4
  Extended EMF Observer/2 -> Mux1/2
  Sliding Mode Observer/1 -> Subsystem1/1(0-2pi)
  Extended EMF Observer/1 -> Subsystem2/1(0-2pi)
  Flux Observer/1 -> Subsystem3/1(0-2pi), Subsystem/1(θ_e)
  Constant/1 -> Sliding Mode Observer/5, Extended EMF Observer/5, Flux Observer/5
  Demux7/2 -> Flux Observer/4
  Demux6/1 -> Flux Observer/1
  Demux7/1 -> Flux Observer/3
  Demux6/2 -> Flux Observer/2
  Demux3/1 -> Sliding Mode Observer/3
  Sliding Mode Observer/2 -> Mux/2
  Flux Observer/2 -> ?
  Demux2/1 -> Sliding Mode Observer/1
  Demux2/2 -> Sliding Mode Observer/2
  Demux3/2 -> Sliding Mode Observer/4

== system FOC/Observer/角度转换 ==
  θ : Inport
  Mux1 : Mux  Inputs=2
  SinCos : Trigonometry  Operator=sincos
  sincos : Outport
  wires:
  Mux1/1 -> sincos/1
  SinCos/2 -> Mux1/2
  θ/1 -> SinCos/1
  SinCos/1 -> Mux1/1

== system FOC/Observer/计算转子反电动势 ==
  Iαβ : Inport
  Uαβ : Inport  Port=2
  Sum5 : Sum  Inputs=+--
  滞后补偿 : DiscreteFilter  Numerator=[0 0 1 1]  Denominator=[2 0 0 0]
  电感分压 : simulink/Discrete/Discrete Derivative  gainval=motor.Ls  ICPrevScaledInput=0.0  OutMin=[]  OutMax=[]  OutDataType=fixdt(1, 16)  OutScaling=2^-10  DoSatur=off
  电阻分压 : Gain  Gain=motor.Rs
  Eαβ : Outport
  tag scope: E_alphabeta=global
  wires:
  Sum5/1 -> [E_alphabeta], Eαβ/1
  滞后补偿/1 -> Sum5/1
  Iαβ/1 -> 电阻分压/1, 电感分压/1
  Uαβ/1 -> 滞后补偿/1
  电阻分压/1 -> Sum5/2
  电感分压/1 -> Sum5/3

== system FOC/Observer/转矩计算 ==
  θ_sincos : Inport
  I_αβ : Inport  Port=2
  Constant : Constant  Value=motor.psi  OutDataTypeStr=single
  Divide1 : Product  Inputs=**
  Gain : Gain  Gain=[-1 1]  Multiplication=Matrix(K*u)
  Gain1 : Gain  Gain=motor.P
  Gain2 : Gain  Gain=1.5
  Product3 : Product
  Unit Delay : UnitDelay  SampleTime=-1
  T : Outport
  wires:
  Gain2/1 -> T/1
  Gain1/1 -> Divide1/2
  θ_sincos/1 -> Unit Delay/1
  I_αβ/1 -> Product3/2
  Unit Delay/1 -> Product3/1
  Gain/1 -> Divide1/1
  Divide1/1 -> Gain2/1
  Constant/1 -> Gain1/1
  Product3/1 -> Gain/1

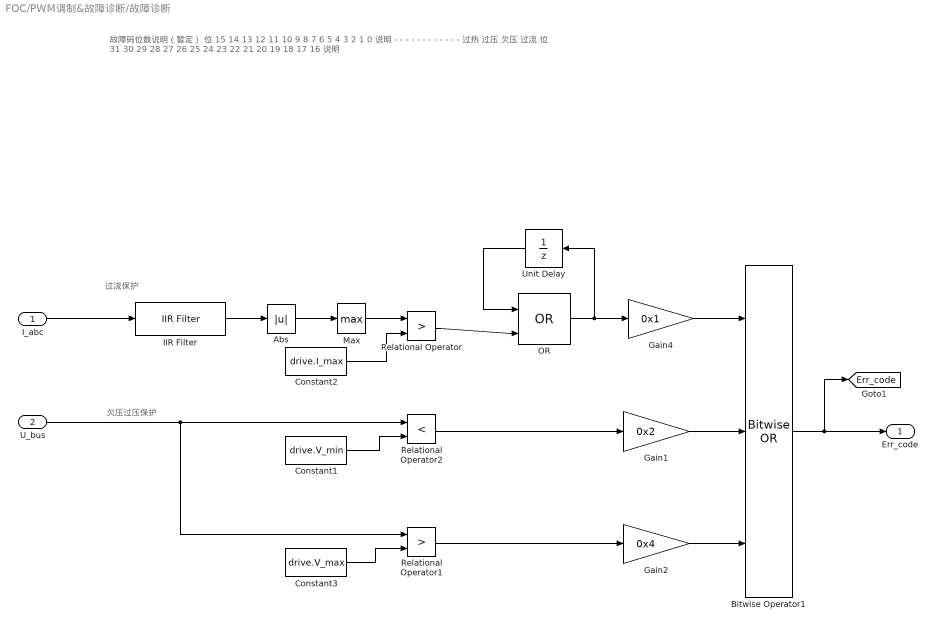
== system FOC/PWM调制&故障诊断/故障诊断 ==
  note: 欠压过压保护
  note: 故障码位数说明（暂定）
      |
      | 位
      | 15
      | 14
      | 13
      | 12
      | 11
      | 10
      | 9
      | 8
      | 7
      | 6
      | 5
      | 4
      | 3
      | 2
      | 1
      | 0
      |
      | 说明
      | -
      | -
      | -
      | -
      | -
      | -
      | -
      | -
      | -
      | -
      | -
      | -
      | 过热
      | 过压
      | 欠压
      | 过流
      |
      | 位
      | 31
      | 30
      | 29
      | 28
      | 27
      | 26
      | 25
      | 24
      | 23
      | 22
      | 21
      | 20
      | 19
      | 18
      | 17
      | 16
      |
      | 说明
      | ​
      | ​
      | ​
      | ​
      | ​
      | ​
      | ​
      | ​
      | ​
      | ​
      | ​
      | ​
      | ​
      | ​
      | ​
      | ​
  note: 过流保护
  I_abc : Inport
  U_bus : Inport  Port=2
  Abs : Abs  SaturateOnIntegerOverflow=off
  Bitwise Operator1 : simulink/Logic and Bit Operations/Bitwise Operator  logicop=OR  UseBitMask=off  NumInputPorts=3  BitMask=bin2dec('11011001')  BitMaskRealWorld=Stored Integer
  Constant1 : Constant  Value=drive.V_min
  Constant2 : Constant  Value=drive.I_max
  Constant3 : Constant  Value=drive.V_max
  Gain1 : Gain  Gain=0x2  OutDataTypeStr=uint32
  Gain2 : Gain  Gain=0x4  OutDataTypeStr=uint32
  Gain4 : Gain  Gain=0x1  OutDataTypeStr=uint32
  IIR Filter : mcbhdlcontrolslib/IIR Filter  VariantControl=Low Pass Filter  VariantSelect=Low-pass  FilterConstantInputType=Specify via dialog  Filter_constant=0.01  advancedSettings=off  Ts=50e-6  cutOff_freq=32.1525
  Max : MinMax  Function=max
  OR : Logic  Operator=OR  IconShape=distinctive  AllPortsSameDT=off  OutDataTypeStr=boolean
  Relational Operator : RelationalOperator  Operator=>  OutDataTypeStr=boolean  RndMeth=Simplest  InputSameDT=off
  Relational Operator1 : RelationalOperator  Operator=>  OutDataTypeStr=boolean  RndMeth=Simplest  InputSameDT=off
  Relational Operator2 : RelationalOperator  Operator=<  OutDataTypeStr=boolean  RndMeth=Simplest  InputSameDT=off
  Unit Delay : UnitDelay  SampleTime=-1
  Err_code : Outport
  tag scope: Err_code=global
  wires:
  OR/1 -> Gain4/1, Unit Delay/1
  Gain4/1 -> Bitwise Operator1/1
  Gain1/1 -> Bitwise Operator1/2
  Gain2/1 -> Bitwise Operator1/3
  Relational Operator/1 -> OR/2
  IIR Filter/1 -> Abs/1
  Bitwise Operator1/1 -> Err_code/1, [Err_code]
  Unit Delay/1 -> OR/1
  Constant3/1 -> Relational Operator1/2
  Relational Operator1/1 -> Gain2/1
  Max/1 -> Relational Operator/1
  Relational Operator2/1 -> Gain1/1
  Constant1/1 -> Relational Operator2/2
  Constant2/1 -> Relational Operator/2
  Abs/1 -> Max/1
  I_abc/1 -> IIR Filter/1
  U_bus/1 -> Relational Operator2/1, Relational Operator1/1

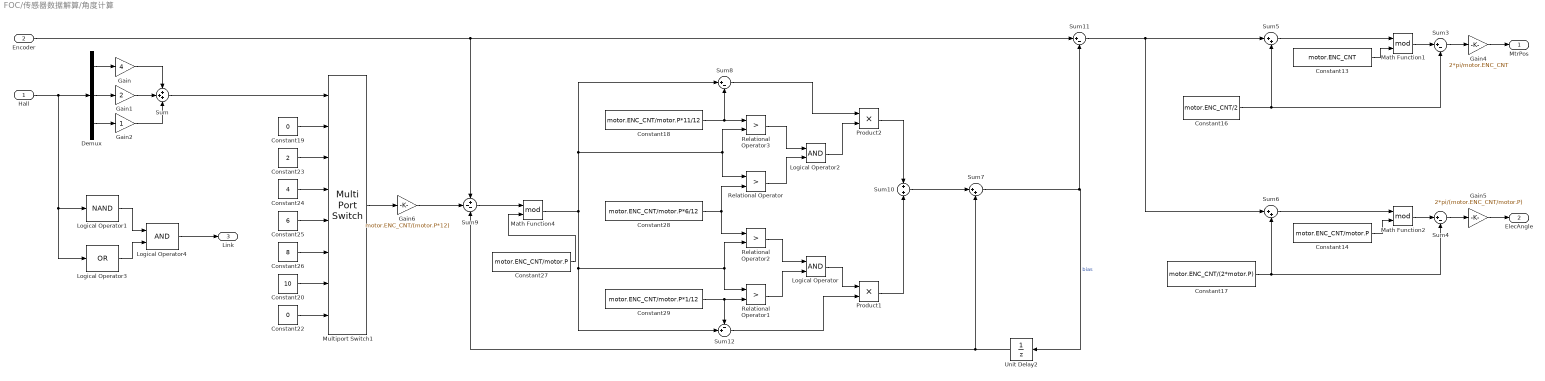
== system FOC/传感器数据解算/角度计算 ==
  Hall : Inport
  Encoder : Inport  Port=2
  Constant13 : Constant  Value=motor.ENC_CNT  OutDataTypeStr=int16
  Constant14 : Constant  Value=motor.ENC_CNT/motor.P  OutDataTypeStr=int16
  Constant16 : Constant  Value=motor.ENC_CNT/2  OutDataTypeStr=int16
  Constant17 : Constant  Value=motor.ENC_CNT/(2*motor.P)  OutDataTypeStr=int16
  Constant18 : Constant  Value=motor.ENC_CNT/motor.P*11/12  OutDataTypeStr=int16
  Constant19 : Constant  Value=0  OutDataTypeStr=int16
  Constant20 : Constant  Value=10  OutDataTypeStr=int16
  Constant22 : Constant  Value=0  OutDataTypeStr=int16
  Constant23 : Constant  Value=2  OutDataTypeStr=int16
  Constant24 : Constant  Value=4  OutDataTypeStr=int16
  Constant25 : Constant  Value=6  OutDataTypeStr=int16
  Constant26 : Constant  Value=8  OutDataTypeStr=int16
  Constant27 : Constant  Value=motor.ENC_CNT/motor.P  OutDataTypeStr=int16
  Constant28 : Constant  Value=motor.ENC_CNT/motor.P*6/12  OutDataTypeStr=int16
  Constant29 : Constant  Value=motor.ENC_CNT/motor.P*1/12  OutDataTypeStr=int16
  Demux : Demux  Outputs=3
  Gain : Gain  Gain=4
  Gain1 : Gain  Gain=2
  Gain2 : Gain
  Gain4 : Gain  Gain=2*pi/motor.ENC_CNT  OutDataTypeStr=single
  Gain5 : Gain  Gain=2*pi/(motor.ENC_CNT/motor.P)  OutDataTypeStr=single
  Gain6 : Gain  Gain=motor.ENC_CNT/(motor.P*12)  OutDataTypeStr=int16
  Logical Operator : Logic  AllPortsSameDT=off  OutDataTypeStr=boolean
  Logical Operator1 : Logic  Operator=NAND  Inputs=1  IconShape=distinctive  AllPortsSameDT=off  OutDataTypeStr=boolean
  Logical Operator2 : Logic  AllPortsSameDT=off  OutDataTypeStr=boolean
  Logical Operator3 : Logic  Operator=OR  Inputs=1  IconShape=distinctive  AllPortsSameDT=off  OutDataTypeStr=boolean
  Logical Operator4 : Logic  IconShape=distinctive  AllPortsSameDT=off  OutDataTypeStr=boolean
  Math Function1 : Math  Operator=mod
  Math Function2 : Math  Operator=mod
  Math Function4 : Math  Operator=mod
  Multiport Switch1 : MultiPortSwitch  DataPortOrder=Specify indices  DataPortIndices={5,4,6,2,3,1}  DataPortForDefault=Additional data port  DiagnosticForDefault=None  SaturateOnIntegerOverflow=off  InputSameDT=off
  Product1 : Product  Inputs=**
  Product2 : Product  Inputs=**
  Relational Operator{,1..3} (4 alike) : RelationalOperator  Operator=>  OutDataTypeStr=boolean  RndMeth=Simplest  InputSameDT=off
  Sum : Sum  Inputs=+++
  Sum10 : Sum  Inputs=+|+
  Sum{3..4,8,11} (4 alike) : Sum  Inputs=|+-
  Sum12 : Sum  Inputs=-+|
  Sum5 : Sum  Inputs=|++
  Sum6 : Sum  Inputs=|++
  Sum7 : Sum  Inputs=|++
  Sum9 : Sum  Inputs=+--
  Unit Delay2 : UnitDelay  SampleTime=-1
  MtrPos : Outport
  ElecAngle : Outport  Port=2
  Link : Outport  Port=3
  wires:
  Sum/1 -> Multiport Switch1/1
  Sum10/1 -> Sum7/1
  Product2/1 -> Sum10/1
  Logical Operator2/1 -> Product2/2
  Encoder/1 -> Sum11/1, Sum9/1
  Relational Operator1/1 -> Logical Operator/2
  Sum7/1 -> Sum11/2, Unit Delay2/1  "bias"
  Constant23/1 -> Multiport Switch1/3
  Sum12/1 -> Product1/2
  Gain6/1 -> Sum9/2
  Math Function4/1 -> Relational Operator1/1, Relational Operator2/2, Sum12/2, Relational Operator3/2, Relational Operator/1, Sum8/1
  Sum8/1 -> Product2/1
  Constant18/1 -> Relational Operator3/1, Sum8/2
  Relational Operator3/1 -> Logical Operator2/1
  Product1/1 -> Sum10/2
  Constant29/1 -> Relational Operator1/2, Sum12/1
  Multiport Switch1/1 -> Gain6/1
  Logical Operator/1 -> Product1/1
  Constant22/1 -> Multiport Switch1/8
  Sum9/1 -> Math Function4/1
  Unit Delay2/1 -> Sum9/3, Sum7/2
  Constant19/1 -> Multiport Switch1/2
  Relational Operator/1 -> Logical Operator2/2
  Constant27/1 -> Math Function4/2
  Constant28/1 -> Relational Operator2/1, Relational Operator/2
  Relational Operator2/1 -> Logical Operator/1
  Constant20/1 -> Multiport Switch1/7
  Constant25/1 -> Multiport Switch1/5
  Constant24/1 -> Multiport Switch1/4
  Constant26/1 -> Multiport Switch1/6
  Logical Operator3/1 -> Logical Operator4/2
  Logical Operator1/1 -> Logical Operator4/1
  Logical Operator4/1 -> Link/1
  Gain2/1 -> Sum/3
  Gain1/1 -> Sum/2
  Demux/3 -> Gain2/1
  Demux/2 -> Gain1/1
  Gain/1 -> Sum/1
  Hall/1 -> Logical Operator1/1, Logical Operator3/1, Demux/1
  Demux/1 -> Gain/1
  Sum4/1 -> Gain5/1
  Constant13/1 -> Math Function1/2
  Sum11/1 -> Sum5/1, Sum6/1
  Constant14/1 -> Math Function2/2
  Sum3/1 -> Gain4/1
  Gain4/1 -> MtrPos/1
  Gain5/1 -> ElecAngle/1
  Math Function1/1 -> Sum3/1
  Math Function2/1 -> Sum4/1
  Constant16/1 -> Sum5/2, Sum3/2
  Constant17/1 -> Sum4/2, Sum6/2
  Sum5/1 -> Math Function1/1
  Sum6/1 -> Math Function2/1

== system FOC/传感器数据解算/转速计算 ==
  note: 五阶巴特沃斯滤波器
  Encoder : Inport
  Constant3 : Constant  Value=motor.ENC_CNT/2  OutDataTypeStr=int16
  Constant4 : Constant  Value=-motor.ENC_CNT/2  OutDataTypeStr=int16
  Difference : simulink/Discrete/Difference  ICPrevInput=0.0  OutMin=[]  OutMax=[]  OutDataType=fixdt(1, 16)  OutScaling=2^-10  DoSatur=off
  Gain : Gain  Gain=2*pi/motor.ENC_CNT  OutDataTypeStr=single
  Gain1 : Gain  Gain=-motor.ENC_CNT  OutDataTypeStr=int16
  Gain2 : Gain  Gain=motor.ENC_CNT  OutDataTypeStr=int16
  Gain3 : Gain  Gain=1/Ts  OutDataTypeStr=single
  IIR Filter{,1..4} (5 alike) : mcbhdlcontrolslib/IIR Filter  VariantControl=Low Pass Filter  VariantSelect=Low-pass  FilterConstantInputType=Specify via dialog  Filter_constant=0.5  advancedSettings=off  Ts=50e-6  cutOff_freq=3183.0989
  Relational Operator : RelationalOperator  Operator=<  RndMeth=Simplest  InputSameDT=off
  Relational Operator1 : RelationalOperator  Operator=<  RndMeth=Simplest  InputSameDT=off
  Sum2 : Sum  Inputs=+++
  MtrSpeed : Outport
  wires:
  IIR Filter4/1 -> MtrSpeed/1
  IIR Filter3/1 -> IIR Filter4/1
  IIR Filter2/1 -> IIR Filter3/1
  Sum2/1 -> Gain3/1
  IIR Filter1/1 -> IIR Filter2/1
  IIR Filter/1 -> IIR Filter1/1
  Relational Operator/1 -> Gain2/1
  Encoder/1 -> Difference/1
  Relational Operator1/1 -> Gain1/1
  Constant4/1 -> Relational Operator/2
  Gain1/1 -> Sum2/1
  Gain3/1 -> Gain/1
  Constant3/1 -> Relational Operator1/1
  Gain/1 -> IIR Filter/1
  Gain2/1 -> Sum2/3
  Difference/1 -> Sum2/2, Relational Operator/1, Relational Operator1/2

== system FOC/全速域电流分配/MJPA ==
  note: $J\left( u_{bus},\omega _m,i_d \right) =-L\frac{{\omega _{mc}}^2}{{\omega _{mc}}^2+{\omega _m}^2}i_d+{Mi_d}^2+\frac{N}{{u_{bus}}^2/3-p_n\omega _m\left( \psi _f+L_di_d \right) ^2}$
  Vbus : Inport
  ω_m : Inport  Port=2
  IIR Filter : mcbhdlcontrolslib/IIR Filter  VariantControl=Low Pass Filter  VariantSelect=Low-pass  FilterConstantInputType=Specify via dialog  Filter_constant=0.1  advancedSettings=off  Ts=50e-6  cutOff_freq=353.6777
  J_function1 : Subsystem  ReferencedSubsystem=J_function
  J_function3 : Subsystem  ReferencedSubsystem=J_function
  Saturation1 : Saturate  UpperLimit=0.1  LowerLimit=-0.1
  Saturation2 : Saturate  UpperLimit=min(motor.I_rated*1.2)  LowerLimit=max(-motor.I_rated*1.2, -motor.psi/motor.Ls)
  Sum2 : Sum  Inputs=|++
  Sum3 : Sum  Inputs=+|-
  Sum4 : Sum  Inputs=|-+
  Unit Delay : UnitDelay  SampleTime=-1
  Δid : Constant  Value=1e-2  OutDataTypeStr=single
  收敛系数 : Gain  Gain=100
  i*_d : Outport
  wires:
  IIR Filter/1 -> i*_d/1
  Saturation2/1 -> Unit Delay/1, IIR Filter/1
  Sum4/1 -> Saturation2/1  "i_d"
  ω_m/1 -> J_function1/2, J_function3/2
  收敛系数/1 -> Saturation1/1
  Vbus/1 -> J_function1/3, J_function3/3
  J_function3/1 -> Sum3/2
  Unit Delay/1 -> J_function3/1, Sum2/2, Sum4/2
  Sum3/1 -> 收敛系数/1  "ΔJ"
  J_function1/1 -> Sum3/1
  Sum2/1 -> J_function1/1
  Δid/1 -> Sum2/1
  Saturation1/1 -> Sum4/1

== system FOC/坐标变换/Subsystem11 ==
  angle : Inport
  Mux : Mux  Inputs=2
  SinCos : Trigonometry  Operator=sincos
  sincos : Outport
  wires:
  angle/1 -> SinCos/1
  SinCos/2 -> Mux/2
  Mux/1 -> sincos/1
  SinCos/1 -> Mux/1

== system FOC/坐标变换/Subsystem2 ==
  αβ : Inport
  sincos : Inport  Port=2
  Demux : Demux  Outputs=2
  Demux1 : Demux  Outputs=2
  Mux : Mux  Inputs=2
  Park Transform : mcbeeMathTransformLib/Clarke to Park Angle Transform  AxisAlignment=D-axis  UseWithEmbedded=on  PhaseInput=Two inputs  ThetaInput=Sine and Cosine electrical position  AngleInput=Per-unit  N_points=1024
  dq : Outport
  wires:
  Park Transform/2 -> Mux/2
  Park Transform/1 -> Mux/1
  Demux1/2 -> Park Transform/4
  αβ/1 -> Demux/1
  Demux1/1 -> Park Transform/3
  Demux/1 -> Park Transform/1
  Mux/1 -> dq/1
  Demux/2 -> Park Transform/2
  sincos/1 -> Demux1/1

== system FOC/坐标变换/Subsystem3 ==
  abc : Inport
  Gain : Gain  Gain=[2/3 -1/3 -1/3;0 sqrt(3)/3 -sqrt(3)/3]  Multiplication=Matrix(K*u)
  αβ : Outport
  wires:
  Gain/1 -> αβ/1
  abc/1 -> Gain/1

== system FOC/坐标变换/Subsystem4 ==
  αβ : Inport
  Demux1 : Demux  Outputs=2
  Gain : Gain  Gain=sqrt(3)/2
  Mux1 : Mux  Inputs=3
  PWM Reference Generator : mcbcontrolslib/PWM Reference Generator  modType=SVM: space vector modulation  inSignal=Valphabeta  expandVoltageInput=on  inputUnits=Per-unit  LimitModulation=off  enableVoltage=on  enableModulationSignal=off  enableDutyCycle=off  expandVoltageOutput=on
  abc : Outport
  wires:
  Gain/1 -> abc/1
  PWM Reference Generator/2 -> Mux1/2
  PWM Reference Generator/1 -> Mux1/1
  PWM Reference Generator/3 -> Mux1/3
  Demux1/2 -> PWM Reference Generator/2
  Demux1/1 -> PWM Reference Generator/1
  Mux1/1 -> Gain/1
  αβ/1 -> Demux1/1

== system FOC/坐标变换/Subsystem5 ==
  dq : Inport
  sincos : Inport  Port=2
  Demux : Demux  Outputs=2
  Demux1 : Demux  Outputs=2
  Inverse Park Transform : mcbeeMathTransformLib/Park to Clarke Angle Transform  AxisAlignment=D-axis  UseWithEmbedded=on  PhaseInput=Two inputs  ThetaInput=Sine and Cosine electrical position  AngleInput=Per-unit  N_points=1024
  Mux : Mux  Inputs=2
  αβ : Outport
  wires:
  Demux1/2 -> Inverse Park Transform/4
  Mux/1 -> αβ/1
  Inverse Park Transform/2 -> Mux/2
  Inverse Park Transform/1 -> Mux/1
  Demux/2 -> Inverse Park Transform/2
  dq/1 -> Demux/1
  Demux/1 -> Inverse Park Transform/1
  Demux1/1 -> Inverse Park Transform/3
  sincos/1 -> Demux1/1
